simulink model "spot410"  (R2024b)
settings: Solver=ode4  StartTime=0.0  StopTime=tsim  FixedStep=baseRate  RelTol=1e-6  AbsTol=1e-6
values from neighbouring files (symbols this model uses):
  baseRate = paramEst(phase,coord).k1    [SpotEstimator.m]
  Gamma1_el = 0.12    [initSpotDefaultParam.m]
  Gamma1_sh = 0.005    [initSpotDefaultParam.m]
  Gamma1_wr = 0.025    [initSpotDefaultParam.m]
  Gamma2_el = 5    [initSpotDefaultParam.m]
  Gamma2_sh = 5    [initSpotDefaultParam.m]
  Gamma2_wr = 5    [initSpotDefaultParam.m]
  Gamma3_el = 10    [initSpotDefaultParam.m]
  Gamma3_sh = 40    [initSpotDefaultParam.m]
  Gamma3_wr = 40    [initSpotDefaultParam.m]
  Gamma4_el = 0.039    [initSpotDefaultParam.m]
  Gamma4_sh = 0.015    [initSpotDefaultParam.m]
  Gamma4_wr = 0.029    [initSpotDefaultParam.m]
  Gamma5_el = 800    [initSpotDefaultParam.m]
  Gamma5_sh = 800    [initSpotDefaultParam.m]
  Gamma5_wr = 800    [initSpotDefaultParam.m]
  Gamma6_el = 0.000001    (= 1e-06)    [initSpotDefaultParam.m]
  Gamma6_sh = 0.005    [initSpotDefaultParam.m]
  Gamma6_wr = 0.02    [initSpotDefaultParam.m]
  Kd_elarm = 0.8    [initSpotDefaultParam.m]
  Kd_sharm = 1.0    (= 1)    [initSpotDefaultParam.m]
  Kd_wrarm = 0.6    [initSpotDefaultParam.m]
  Kp_elarm = 1.2    [initSpotDefaultParam.m]
  Kp_sharm = 1.5    [initSpotDefaultParam.m]
  Kp_wrarm = 1.0    (= 1)    [initSpotDefaultParam.m]
  PWMFreq = 5    [initSpotDefaultParam.m]
  Tz_lim_elarm = .1    (= 0.1)    [initSpotDefaultParam.m]
  Tz_lim_sharm = .1    (= 0.1)    [initSpotDefaultParam.m]
  Tz_lim_wrarm = .1    (= 0.1)    [initSpotDefaultParam.m]
undefined symbols (not defined in the file or in its folder): a1, a2, a3, b0, b1, b2, b3, dataRate, DiscIntNeverNeededParam, drop_states_ARM, drop_states_BLACK, drop_states_BLUE, drop_states_RED, F_black_X_nominal, F_black_Y_nominal, F_blue_X_nominal, F_blue_Y_nominal, F_red_X_nominal, F_red_Y_nominal, F_thrusters_BLACK, F_thrusters_BLUE, F_thrusters_RED, home_states_BLACK, home_states_BLUE, home_states_RED, IBLACK, IBLUE, IDIST, IEE, init_states_BLACK, init_states_BLUE, init_states_RED, IPROX, IRED, K_BLACK, K_BLUE, K_RED, Kd_tb, Kd_tblue, Kd_tr, Kd_xb, Kd_xblue, Kd_xr, Kd_yb, Kd_yblue, Kd_yr, Kp_tb, Kp_tblue, Kp_tr, Kp_xb, Kp_xblue, Kp_xr, Kp_yb, Kp_yblue, Kp_yr, mBLACK, mBLUE, mDIST, mEE, mPROX ... (+21)
libraries: simulink x30, nvidiaSharedBlocks x19, MainLibrary x5, dspinverses x3, nvidiaIMUSensorslib x1
(part 4 of 8)

== system spot410/1 - Experiment Logic/Phase #3: Experiment/Sub-Phase #2  ==
  note: Experiment Logic (BLACK)
  note: Experiment Logic (Robotic Manipulator)
  note: Experiment Logic (BLUE)
  note: Experiment Logic (RED)
  note: Control Blocks
  Action Port : ActionPort  ActionPortLabel=elseif((u1 < u3 & u1 >= u2))
  Constant{11..12,14..15,18} (5 alike) : Constant  Value=0
  Constant4 : Constant  Value=2
  Constant5 : Constant  Value=2
  Constant6 : Constant
  Constant8 : Constant  Value=2
  Data Store Write1 : DataStoreWrite  DataStoreName=ARM_Path_Planner_Selection  IndexOptions=Index vector (dialog)  Indices=1  OutputSizes=1
  Data Store Write13 : DataStoreWrite  DataStoreName=ARM_Desired_States  IndexOptions=Index vector (dialog)  Indices=1  OutputSizes=1
  Data Store Write16 : DataStoreWrite  DataStoreName=BLUE_Control_Law_Enabler  IndexOptions=Index vector (dialog)  Indices=1  OutputSizes=1
  Data Store Write18 : DataStoreWrite  DataStoreName=BLUE_Desired_States  IndexOptions=Index vector (dialog)  Indices=1  OutputSizes=1
  Data Store Write2 : DataStoreWrite  DataStoreName=ARM_Control_Law_Enabler  IndexOptions=Index vector (dialog)  Indices=1  OutputSizes=1
  Data Store Write22 : DataStoreWrite  DataStoreName=BLUE_Path_Planner_Selection  IndexOptions=Index vector (dialog)  Indices=1  OutputSizes=1
  Data Store Write23 : DataStoreWrite  DataStoreName=BLACK_Path_Planner_Selection  IndexOptions=Index vector (dialog)  Indices=1  OutputSizes=1
  Data Store Write24 : DataStoreWrite  DataStoreName=RED_Path_Planner_Selection  IndexOptions=Index vector (dialog)  Indices=1  OutputSizes=1
  Data Store Write3 : DataStoreWrite  DataStoreName=RED_Control_Law_Enabler  IndexOptions=Index vector (dialog)  Indices=1  OutputSizes=1
  Data Store Write4 : DataStoreWrite  DataStoreName=BLACK_Control_Law_Enabler  IndexOptions=Index vector (dialog)  Indices=1  OutputSizes=1
  Data Store Write5 : DataStoreWrite  DataStoreName=BLACK_Desired_States  IndexOptions=Index vector (dialog)  Indices=1  OutputSizes=1
  Data Store Write7 : DataStoreWrite  DataStoreName=Float_State  IndexOptions=Index vector (dialog)  Indices=1  OutputSizes=1
  Data Store Write9 : DataStoreWrite  DataStoreName=RED_Desired_States  IndexOptions=Index vector (dialog)  Indices=1  OutputSizes=1
  Desired Joint Angles RED : Subsystem
  Desired Position BLACK : Subsystem
  Desired Position BLUE : Subsystem
  Desired Position RED : Subsystem
  wires:
  Desired Position RED/1(Target Array) -> Data Store Write9/1
  Desired Position BLACK/1(Target Array) -> Data Store Write5/1
  Desired Position BLUE/1(Target Array) -> Data Store Write18/1
  Constant12/1 -> Data Store Write1/1
  Constant18/1 -> Data Store Write2/1
  Constant6/1 -> Data Store Write7/1
  Constant15/1 -> Data Store Write22/1
  Constant14/1 -> Data Store Write23/1
  Constant5/1 -> Data Store Write3/1
  Constant11/1 -> Data Store Write24/1
  Constant8/1 -> Data Store Write16/1
  Constant4/1 -> Data Store Write4/1
  Desired Joint Angles RED/1(Target Array) -> Data Store Write13/1

== system spot410/1 - Experiment Logic/Phase #3: Experiment/Sub-Phase #3  ==
  note: Experiment Logic (BLACK)
  note: Experiment Logic (Robotic Manipulator)
  note: Experiment Logic (BLUE)
  note: Experiment Logic (RED)
  note: Control Blocks
  Action Port : ActionPort  ActionPortLabel=elseif((u1 < u4 & u1 >= u3))
  Constant{11..12,14..15,18} (5 alike) : Constant  Value=0
  Constant4 : Constant  Value=2
  Constant5 : Constant  Value=2
  Constant6 : Constant
  Constant8 : Constant  Value=2
  Data Store Write1 : DataStoreWrite  DataStoreName=ARM_Path_Planner_Selection  IndexOptions=Index vector (dialog)  Indices=1  OutputSizes=1
  Data Store Write13 : DataStoreWrite  DataStoreName=ARM_Desired_States  IndexOptions=Index vector (dialog)  Indices=1  OutputSizes=1
  Data Store Write16 : DataStoreWrite  DataStoreName=BLUE_Control_Law_Enabler  IndexOptions=Index vector (dialog)  Indices=1  OutputSizes=1
  Data Store Write18 : DataStoreWrite  DataStoreName=BLUE_Desired_States  IndexOptions=Index vector (dialog)  Indices=1  OutputSizes=1
  Data Store Write2 : DataStoreWrite  DataStoreName=ARM_Control_Law_Enabler  IndexOptions=Index vector (dialog)  Indices=1  OutputSizes=1
  Data Store Write22 : DataStoreWrite  DataStoreName=BLUE_Path_Planner_Selection  IndexOptions=Index vector (dialog)  Indices=1  OutputSizes=1
  Data Store Write23 : DataStoreWrite  DataStoreName=BLACK_Path_Planner_Selection  IndexOptions=Index vector (dialog)  Indices=1  OutputSizes=1
  Data Store Write24 : DataStoreWrite  DataStoreName=RED_Path_Planner_Selection  IndexOptions=Index vector (dialog)  Indices=1  OutputSizes=1
  Data Store Write3 : DataStoreWrite  DataStoreName=RED_Control_Law_Enabler  IndexOptions=Index vector (dialog)  Indices=1  OutputSizes=1
  Data Store Write4 : DataStoreWrite  DataStoreName=BLACK_Control_Law_Enabler  IndexOptions=Index vector (dialog)  Indices=1  OutputSizes=1
  Data Store Write5 : DataStoreWrite  DataStoreName=BLACK_Desired_States  IndexOptions=Index vector (dialog)  Indices=1  OutputSizes=1
  Data Store Write7 : DataStoreWrite  DataStoreName=Float_State  IndexOptions=Index vector (dialog)  Indices=1  OutputSizes=1
  Data Store Write9 : DataStoreWrite  DataStoreName=RED_Desired_States  IndexOptions=Index vector (dialog)  Indices=1  OutputSizes=1
  Desired Joint Angles RED : Subsystem
  Desired Position BLACK : Subsystem
  Desired Position BLUE : Subsystem
  Desired Position RED : Subsystem
  wires:
  Desired Position RED/1(Target Array) -> Data Store Write9/1
  Desired Position BLACK/1(Target Array) -> Data Store Write5/1
  Desired Position BLUE/1(Target Array) -> Data Store Write18/1
  Desired Joint Angles RED/1(Target Array) -> Data Store Write13/1
  Constant12/1 -> Data Store Write1/1
  Constant18/1 -> Data Store Write2/1
  Constant6/1 -> Data Store Write7/1
  Constant15/1 -> Data Store Write22/1
  Constant14/1 -> Data Store Write23/1
  Constant5/1 -> Data Store Write3/1
  Constant11/1 -> Data Store Write24/1
  Constant8/1 -> Data Store Write16/1
  Constant4/1 -> Data Store Write4/1

== system spot410/1 - Experiment Logic/Phase #3: Experiment/Sub-Phase #4 ==
  note: Experiment Logic (BLACK)
  note: Experiment Logic (Robotic Manipulator)
  note: Experiment Logic (BLUE)
  note: Experiment Logic (RED)
  note: Control Blocks
  Action Port : ActionPort  ActionPortLabel=elseif( (u1 < u5 & u1 >= u4))
  Constant{11..12,14..15,18} (5 alike) : Constant  Value=0
  Constant4 : Constant  Value=2
  Constant5 : Constant  Value=2
  Constant6 : Constant
  Constant8 : Constant  Value=2
  Data Store Write1 : DataStoreWrite  DataStoreName=ARM_Path_Planner_Selection  IndexOptions=Index vector (dialog)  Indices=1  OutputSizes=1
  Data Store Write13 : DataStoreWrite  DataStoreName=ARM_Desired_States  IndexOptions=Index vector (dialog)  Indices=1  OutputSizes=1
  Data Store Write16 : DataStoreWrite  DataStoreName=BLUE_Control_Law_Enabler  IndexOptions=Index vector (dialog)  Indices=1  OutputSizes=1
  Data Store Write18 : DataStoreWrite  DataStoreName=BLUE_Desired_States  IndexOptions=Index vector (dialog)  Indices=1  OutputSizes=1
  Data Store Write2 : DataStoreWrite  DataStoreName=ARM_Control_Law_Enabler  IndexOptions=Index vector (dialog)  Indices=1  OutputSizes=1
  Data Store Write22 : DataStoreWrite  DataStoreName=BLUE_Path_Planner_Selection  IndexOptions=Index vector (dialog)  Indices=1  OutputSizes=1
  Data Store Write23 : DataStoreWrite  DataStoreName=BLACK_Path_Planner_Selection  IndexOptions=Index vector (dialog)  Indices=1  OutputSizes=1
  Data Store Write24 : DataStoreWrite  DataStoreName=RED_Path_Planner_Selection  IndexOptions=Index vector (dialog)  Indices=1  OutputSizes=1
  Data Store Write3 : DataStoreWrite  DataStoreName=RED_Control_Law_Enabler  IndexOptions=Index vector (dialog)  Indices=1  OutputSizes=1
  Data Store Write4 : DataStoreWrite  DataStoreName=BLACK_Control_Law_Enabler  IndexOptions=Index vector (dialog)  Indices=1  OutputSizes=1
  Data Store Write5 : DataStoreWrite  DataStoreName=BLACK_Desired_States  IndexOptions=Index vector (dialog)  Indices=1  OutputSizes=1
  Data Store Write7 : DataStoreWrite  DataStoreName=Float_State  IndexOptions=Index vector (dialog)  Indices=1  OutputSizes=1
  Data Store Write9 : DataStoreWrite  DataStoreName=RED_Desired_States  IndexOptions=Index vector (dialog)  Indices=1  OutputSizes=1
  Desired Joint Angles RED : Subsystem
  Desired Position BLACK : Subsystem
  Desired Position BLUE : Subsystem
  Desired Position RED : Subsystem
  wires:
  Desired Position RED/1(Target Array) -> Data Store Write9/1
  Desired Position BLACK/1(Target Array) -> Data Store Write5/1
  Desired Position BLUE/1(Target Array) -> Data Store Write18/1
  Desired Joint Angles RED/1(Target Array) -> Data Store Write13/1
  Constant12/1 -> Data Store Write1/1
  Constant18/1 -> Data Store Write2/1
  Constant6/1 -> Data Store Write7/1
  Constant15/1 -> Data Store Write22/1
  Constant14/1 -> Data Store Write23/1
  Constant5/1 -> Data Store Write3/1
  Constant11/1 -> Data Store Write24/1
  Constant8/1 -> Data Store Write16/1
  Constant4/1 -> Data Store Write4/1

== system spot410/1 - Experiment Logic/Phase #4: Return Home/Desired Joint Angles RED ==
  Constant1 : Constant  Value=pi/2
  Constant2 : Constant  Value=0
  Constant3 : Constant  Value=pi/2
  Mux : Mux  Inputs=3
  Target Array : Outport
  wires:
  Mux/1 -> Target Array/1
  Constant3/1 -> Mux/1
  Constant1/1 -> Mux/2
  Constant2/1 -> Mux/3

== system spot410/1 - Experiment Logic/Phase #4: Return Home/Desired Position BLACK ==
  Desired States (BLACK) : Constant  Value=home_states_BLACK  SampleTime=-1
  Target Array : Outport
  wires:
  Desired States (BLACK)/1 -> Target Array/1

== system spot410/1 - Experiment Logic/Phase #4: Return Home/Desired Position BLUE ==
  Desired States (BLUE) : Constant  Value=home_states_BLUE  SampleTime=-1
  Target Array : Outport
  wires:
  Desired States (BLUE)/1 -> Target Array/1

== system spot410/1 - Experiment Logic/Phase #4: Return Home/Desired Position RED ==
  Constant2 : Constant  Value=home_states_RED
  Target Array : Outport
  wires:
  Constant2/1 -> Target Array/1

== system spot410/1 - Experiment Logic/Phase #5: Hold Home/Desired Joint Angles RED ==
  Constant1 : Constant  Value=pi/2
  Constant2 : Constant  Value=0
  Constant3 : Constant  Value=pi/2
  Mux : Mux  Inputs=3
  Target Array : Outport
  wires:
  Mux/1 -> Target Array/1
  Constant3/1 -> Mux/1
  Constant1/1 -> Mux/2
  Constant2/1 -> Mux/3

== system spot410/1 - Experiment Logic/Phase #5: Hold Home/Desired Position BLACK ==
  Desired States (BLACK) : Constant  Value=home_states_BLACK  SampleTime=-1
  Target Array : Outport
  wires:
  Desired States (BLACK)/1 -> Target Array/1

== system spot410/1 - Experiment Logic/Phase #5: Hold Home/Desired Position BLUE ==
  Desired States (BLUE) : Constant  Value=home_states_BLUE  SampleTime=-1
  Target Array : Outport
  wires:
  Desired States (BLUE)/1 -> Target Array/1

== system spot410/1 - Experiment Logic/Phase #5: Hold Home/Desired Position RED ==
  Constant2 : Constant  Value=home_states_RED
  Target Array : Outport
  wires:
  Constant2/1 -> Target Array/1

== system spot410/2 - Guidance/Custom PPL (ARM)/Desired Position ==
  Data Store Read : DataStoreRead  DataStoreName=ARM_Desired_States  IndexOptions=Index vector (dialog)  Indices=1  OutputSizes=1
  Position Array : Outport
  wires:
  Data Store Read/1 -> Position Array/1

== system spot410/2 - Guidance/Custom PPL (BLACK)/Desired Position ==
  BLACK_Px : DataStoreRead  DataStoreName=BLACK_Desired_States  IndexOptions=Index vector (dialog)  Indices=1  OutputSizes=1
  Position Array : Outport
  wires:
  BLACK_Px/1 -> Position Array/1

== system spot410/2 - Guidance/Custom PPL (BLUE)/Desired Position ==
  Data Store Read4 : DataStoreRead  DataStoreName=BLUE_Desired_States  IndexOptions=Index vector (dialog)  Indices=1  OutputSizes=1
  Position Array : Outport
  wires:
  Data Store Read4/1 -> Position Array/1

== system spot410/2 - Guidance/Custom PPL (RED)/Desired Position ==
  RED_Px : DataStoreRead  DataStoreName=RED_Desired_States  IndexOptions=Index vector (dialog)  Indices=1  OutputSizes=1
  Position Array : Outport
  wires:
  RED_Px/1 -> Position Array/1

== system spot410/2 - Guidance/Default APF PPL (BLACK)/Current Position RED ==
  Demux : Demux  Outputs=[3,6]
  RED_Px : DataStoreRead  DataStoreName=BLACK_Measured_States  IndexOptions=Index vector (dialog)  Indices=1  OutputSizes=1
  Terminator : Terminator
  Position Array : Outport
  wires:
  RED_Px/1 -> Demux/1
  Demux/1 -> Position Array/1
  Demux/2 -> Terminator/1

== system spot410/2 - Guidance/Default APF PPL (BLACK)/Obstacles ==
  Current Position BLUE : Subsystem
  Current Position RED : Subsystem
  Matrix Concatenate : Concatenate  Mode=Multidimensional array
  Obstacle Positions : Outport
  wires:
  Current Position RED/1(Position Array) -> Matrix Concatenate/2
  Current Position BLUE/1(Position Array) -> Matrix Concatenate/1
  Matrix Concatenate/1 -> Obstacle Positions/1

== system spot410/2 - Guidance/Default APF PPL (RED)/Current Position RED ==
  Demux : Demux  Outputs=[3,6]
  RED_Px : DataStoreRead  DataStoreName=RED_Measured_States  IndexOptions=Index vector (dialog)  Indices=1  OutputSizes=1
  Terminator : Terminator
  Position Array : Outport
  wires:
  RED_Px/1 -> Demux/1
  Demux/1 -> Position Array/1
  Demux/2 -> Terminator/1

== system spot410/2 - Guidance/Default APF PPL (RED)/Obstacles ==
  Current Position BLACK : Subsystem
  Current Position BLUE : Subsystem
  Matrix Concatenate : Concatenate  Mode=Multidimensional array
  Obstacle Positions : Outport
  wires:
  Current Position BLACK/1(Position Array) -> Matrix Concatenate/2
  Current Position BLUE/1(Position Array) -> Matrix Concatenate/1
  Matrix Concatenate/1 -> Obstacle Positions/1

== system spot410/2 - Guidance/Disable PPL (ARM)/Desired Position ==
  Data Store Read : DataStoreRead  DataStoreName=ARM_Desired_States  IndexOptions=Index vector (dialog)  Indices=1  OutputSizes=1
  Position Array : Outport
  wires:
  Data Store Read/1 -> Position Array/1

== system spot410/2 - Guidance/Disable PPL (BLACK)/Desired Position ==
  BLACK_Px : DataStoreRead  DataStoreName=BLACK_Desired_States  IndexOptions=Index vector (dialog)  Indices=1  OutputSizes=1
  Position Array : Outport
  wires:
  BLACK_Px/1 -> Position Array/1

== system spot410/2 - Guidance/Disable PPL (BLUE)/Desired Position ==
  Data Store Read4 : DataStoreRead  DataStoreName=BLUE_Desired_States  IndexOptions=Index vector (dialog)  Indices=1  OutputSizes=1
  Position Array : Outport
  wires:
  Data Store Read4/1 -> Position Array/1

== system spot410/2 - Guidance/Disable PPL (RED)/Desired Position ==
  RED_Px : DataStoreRead  DataStoreName=RED_Desired_States  IndexOptions=Index vector (dialog)  Indices=1  OutputSizes=1
  Position Array : Outport
  wires:
  RED_Px/1 -> Position Array/1

== system spot410/3 - Control/Default LQR Control (BLACK)/Calculate Error ==
  Desired Attitude : Inport
  Measured Attitude : Inport  Port=2
  MATLAB Function : MATLAB Function  TreatAsAtomicUnit=on
  Attitude Error : Outport
  wires:
  MATLAB Function/1(Rz_error) -> Attitude Error/1
  Desired Attitude/1 -> MATLAB Function/1(Rz_path)
  Measured Attitude/1 -> MATLAB Function/2(Rz_measured)

== system spot410/3 - Control/Default LQR Control (BLUE)/Calculate Error ==
  Desired Attitude : Inport
  Measured Attitude : Inport  Port=2
  MATLAB Function : MATLAB Function  TreatAsAtomicUnit=on
  Attitude Error : Outport
  wires:
  MATLAB Function/1(Rz_error) -> Attitude Error/1
  Desired Attitude/1 -> MATLAB Function/1(Rz_path)
  Measured Attitude/1 -> MATLAB Function/2(Rz_measured)

== system spot410/3 - Control/Default LQR Control (RED)/Calculate Error ==
  Desired Attitude : Inport
  Measured Attitude : Inport  Port=2
  MATLAB Function : MATLAB Function  TreatAsAtomicUnit=on
  Attitude Error : Outport
  wires:
  MATLAB Function/1(Rz_error) -> Attitude Error/1
  Desired Attitude/1 -> MATLAB Function/1(Rz_path)
  Measured Attitude/1 -> MATLAB Function/2(Rz_measured)

== system spot410/3 - Control/Default PD (ARM)/Passthrough for Experiment ==
  q1_desired : Inport
  q2_desired : Inport  Port=2
  q3_desired : Inport  Port=3
  Action Port : ActionPort  ActionPortLabel=else
  q1_command : Outport
  q2_command : Outport  Port=2
  q3_command : Outport  Port=3
  wires:
  q3_desired/1 -> q3_command/1
  q1_desired/1 -> q1_command/1
  q2_desired/1 -> q2_command/1

== system spot410/3 - Control/Default PD (ARM)/Simulated Position Controller ==
  q1_desired : Inport
  q2_desired : Inport  Port=2
  q3_desired : Inport  Port=3
  Action Port : ActionPort  ActionPortLabel=if(u1 == 1)
  Custom Discrete PD (Elbow) : Subsystem
  Custom Discrete PD (Shoulder) : Subsystem
  Custom Discrete PD (Wrist) : Subsystem
  Data Store Read2 : DataStoreRead  DataStoreName=ARM_Measured_States  IndexOptions=Index vector (dialog)  Indices=1  OutputSizes=1
  Demux : Demux  Outputs=[1,1,1,3]
  Saturation : Saturate  UpperLimit=Tz_lim_sharm  LowerLimit=-Tz_lim_sharm
  Saturation1 : Saturate  UpperLimit=Tz_lim_elarm  LowerLimit=-Tz_lim_elarm
  Saturation3 : Saturate  UpperLimit=Tz_lim_wrarm  LowerLimit=-Tz_lim_wrarm
  Subtract2 : Sum  Inputs=+-
  Subtract3 : Sum  Inputs=+-
  Subtract4 : Sum  Inputs=+-
  Terminator : Terminator
  q1_command : Outport
  q2_command : Outport  Port=2
  q3_command : Outport  Port=3
  wires:
  Saturation3/1 -> q3_command/1
  Subtract4/1 -> Custom Discrete PD (Wrist)/1(ey)
  Custom Discrete PD (Shoulder)/1(Fx) -> Saturation/1
  Custom Discrete PD (Elbow)/1(Fy) -> Saturation1/1
  Saturation/1 -> q1_command/1
  Subtract2/1 -> Custom Discrete PD (Shoulder)/1(ex)
  Saturation1/1 -> q2_command/1
  Custom Discrete PD (Wrist)/1(Fy) -> Saturation3/1
  Subtract3/1 -> Custom Discrete PD (Elbow)/1(ey)
  Demux/1 -> Subtract2/2
  Demux/2 -> Subtract3/2
  Demux/3 -> Subtract4/2
  q1_desired/1 -> Subtract2/1
  q2_desired/1 -> Subtract3/1
  q3_desired/1 -> Subtract4/1
  Data Store Read2/1 -> Demux/1
  Demux/4 -> Terminator/1

== system spot410/3 - Control/Default PD Control (BLACK)/Calculate Error ==
  Desired Attitude : Inport
  Measured Attitude : Inport  Port=2
  MATLAB Function : MATLAB Function  TreatAsAtomicUnit=on
  Attitude Error : Outport
  wires:
  MATLAB Function/1(Rz_error) -> Attitude Error/1
  Desired Attitude/1 -> MATLAB Function/1(Rz_path)
  Measured Attitude/1 -> MATLAB Function/2(Rz_measured)

== system spot410/3 - Control/Default PD Control (BLUE)/Calculate Error ==
  Desired Attitude : Inport
  Measured Attitude : Inport  Port=2
  MATLAB Function : MATLAB Function  TreatAsAtomicUnit=on
  Attitude Error : Outport
  wires:
  MATLAB Function/1(Rz_error) -> Attitude Error/1
  Desired Attitude/1 -> MATLAB Function/1(Rz_path)
  Measured Attitude/1 -> MATLAB Function/2(Rz_measured)

== system spot410/3 - Control/Default PD Control (RED)/Calculate Error ==
  Desired Attitude : Inport
  Measured Attitude : Inport  Port=2
  MATLAB Function : MATLAB Function  TreatAsAtomicUnit=on
  Attitude Error : Outport
  wires:
  MATLAB Function/1(Rz_error) -> Attitude Error/1
  Desired Attitude/1 -> MATLAB Function/1(Rz_path)
  Measured Attitude/1 -> MATLAB Function/2(Rz_measured)

== system spot410/PhaseSpace Camera Code/Use Hardware to Obtain States/Receive and Process Phasespace Data ==
  "Adjust Time " : Subsystem
  Check for Sychronization : Subsystem
  Clock : Clock
  Demux2 : Demux  Outputs=[1,18]
  Mux : Mux  Inputs=2
  Receive PhaseSpace Data : nvidiaSharedBlocks/UDP Receive  localURL='0.0.0.0'  localPort=31534  remoteURL='0.0.0.0'  remotePort=-1  recvBufferSize=8192  signalDatatype=double  dims=19  isVarSize=off  showBlockingTime=off  blockingTime=0  sampletime=-1  blockPlatform=NVIDIA
  Reshape : Reshape  OutputDimensionality=Customize  OutputDimensions=[19,1]
  Terminator : Terminator
  PhaseSpace Data : Outport
  PhaseSpace Clock : Outport  Port=2
  wires:
  Check for Sychronization/1(StartClock) -> "Adjust Time "/1(ClockStart)
  Reshape/1 -> Demux2/1
  "Adjust Time "/1(ClockAdjusted) -> Mux/1
  Demux2/2 -> Mux/2
  Mux/1 -> PhaseSpace Data/1
  Receive PhaseSpace Data/2 -> Terminator/1
  Receive PhaseSpace Data/1 -> Reshape/1
  Clock/1 -> "Adjust Time "/2(ClockRaw)
  Demux2/1 -> PhaseSpace Clock/1

== system spot410/PhaseSpace Camera Code/Use Hardware to Obtain States/Store BLACK Data ==
  note: Store BLACK Positions and Velocities
  BLACK Data : Inport
  BLACK Velocities : Inport  Port=2
  PS Clock : Inport  Port=3
  Calculate True Time Step : Subsystem
      settings: PortSchema="{\"entries\":[{\"content\":{\"sides\":[{\"content\":{\"connectorIds\":[\"In1\"]},\"type\":\"ConnectorPlacement.EquallySpacedRectSide\",\"uuid\":\"62932c5c-f2a7-44c8-96b4-4a75bab3a126\"},{\"content\":{\"connectorIds\":[\"Out1\"],\"side\":\"RIGHT\"},\"type\":\"ConnectorPlacement.EquallySpacedRectSide\",\"uuid\":\"82b3b717-2171-4047-b0df-3cd41cf9dfc7\"},{\"content\":{\"side\":\"TOP\"},\"type\":\"ConnectorPlacement.EquallySpacedRectSide\",\"uuid\":\"a142272a-a0ff-4882-8a2d-4633b3c7e02f\"},{\"content\":{\"connectorIds\":[\"In2\"],\"side\":\"BOTTOM\"},\"type\":\"ConnectorPlacement.EquallySpacedRectSide\",\"uuid\":\"b1e1ff4c-66d6-488f-92fb-77f76780833b\"}]},\"type\":\"ConnectorPlacement.EquallySpacedConnector\",\"uuid\":\"98c51868-8a10-4b52-aae4-56f6042c65c4\"}],\"packageUris\":[\"http://schema.mathworks.com/mf0/Connector/R2020b\"],\"version\":\"1.0\"}"
  Convert BLACKVX from [mm] to [m] : Gain  Gain=1/1000
  Convert BLACKVY from [mm] to [m] : Gain  Gain=1/1000
  Convert BLAX from [mm] to [m] : Gain  Gain=1/1000
  Convert BLAY from [mm] to [m] : Gain  Gain=1/1000
  Demux : Demux  Outputs=3
  Demux2 : Demux  Outputs=3
  Demux3 : Demux  Outputs=3
  Mux{1..4} (4 alike) : Mux  Inputs=3
  RED_Px7 : DataStoreWrite  DataStoreName=BLACK_Measured_States  IndexOptions=Index vector (dialog)  Indices=1  OutputSizes=1
  Reshape : Reshape  OutputDimensionality=Column vector (2-D)
  Subsystem1 : Subsystem
  Subsystem2 : Subsystem
  Wrap : Subsystem
  wires:
  Demux3/1 -> Convert BLAX from [mm] to [m]/1
  Demux3/2 -> Convert BLAY from [mm] to [m]/1
  BLACK Data/1 -> Demux3/1
  Demux/3 -> Wrap/1(Unwrapped Angle)
  Reshape/1 -> Subsystem1/2(y)
  Demux/1 -> Mux1/1
  Convert BLAY from [mm] to [m]/1 -> Mux3/2
  Calculate True Time Step/1(dt_out) -> Subsystem2/1(dt), Subsystem1/1(dt)
  Mux3/1 -> Subsystem2/2(y), Demux/1, Calculate True Time Step/2(Data)
  Wrap/1(Wrapped Angle) -> Mux1/3
  Convert BLAX from [mm] to [m]/1 -> Mux3/1
  Mux2/1 -> RED_Px7/1
  Demux/2 -> Mux1/2
  Subsystem2/1(dy/dt) -> Reshape/1
  PS Clock/1 -> Calculate True Time Step/1(Time)
  Demux3/3 -> Mux3/3
  Mux1/1 -> Mux2/1
  Subsystem1/1(dy/dt) -> Mux2/3
  BLACK Velocities/1 -> Demux2/1
  Demux2/3 -> Mux4/3
  Convert BLACKVX from [mm] to [m]/1 -> Mux4/1
  Convert BLACKVY from [mm] to [m]/1 -> Mux4/2
  Mux4/1 -> Mux2/2
  Demux2/2 -> Convert BLACKVY from [mm] to [m]/1
  Demux2/1 -> Convert BLACKVX from [mm] to [m]/1

== system spot410/PhaseSpace Camera Code/Use Hardware to Obtain States/Store BLUE Data ==
  note: Store BLUE Positions and Velocities
  BLUE Data : Inport
  BLUE Velocities : Inport  Port=2
  PS Clock : Inport  Port=3
  Calculate True Time Step : Subsystem
      settings: PortSchema="{\"entries\":[{\"content\":{\"sides\":[{\"content\":{\"connectorIds\":[\"In1\"]},\"type\":\"ConnectorPlacement.EquallySpacedRectSide\",\"uuid\":\"62932c5c-f2a7-44c8-96b4-4a75bab3a126\"},{\"content\":{\"connectorIds\":[\"Out1\"],\"side\":\"RIGHT\"},\"type\":\"ConnectorPlacement.EquallySpacedRectSide\",\"uuid\":\"82b3b717-2171-4047-b0df-3cd41cf9dfc7\"},{\"content\":{\"side\":\"TOP\"},\"type\":\"ConnectorPlacement.EquallySpacedRectSide\",\"uuid\":\"a142272a-a0ff-4882-8a2d-4633b3c7e02f\"},{\"content\":{\"connectorIds\":[\"In2\"],\"side\":\"BOTTOM\"},\"type\":\"ConnectorPlacement.EquallySpacedRectSide\",\"uuid\":\"b1e1ff4c-66d6-488f-92fb-77f76780833b\"}]},\"type\":\"ConnectorPlacement.EquallySpacedConnector\",\"uuid\":\"98c51868-8a10-4b52-aae4-56f6042c65c4\"}],\"packageUris\":[\"http://schema.mathworks.com/mf0/Connector/R2020b\"],\"version\":\"1.0\"}"
  Convert BLUEVX from [mm] to [m] : Gain  Gain=1/1000
  Convert BLUEVY from [mm] to [m] : Gain  Gain=1/1000
  Convert BLUX from [mm] to [m] : Gain  Gain=1/1000
  Convert BLUY from [mm] to [m] : Gain  Gain=1/1000
  Demux : Demux  Outputs=3
  Demux2 : Demux  Outputs=3
  Demux5 : Demux  Outputs=3
  Mux{1..4} (4 alike) : Mux  Inputs=3
  RED_Px7 : DataStoreWrite  DataStoreName=BLUE_Measured_States  IndexOptions=Index vector (dialog)  Indices=1  OutputSizes=1
  Reshape : Reshape  OutputDimensionality=Column vector (2-D)
  Subsystem1 : Subsystem
  Subsystem2 : Subsystem
  Wrap : Subsystem
  wires:
  Demux5/2 -> Convert BLUY from [mm] to [m]/1
  Demux5/1 -> Convert BLUX from [mm] to [m]/1
  BLUE Data/1 -> Demux5/1
  Calculate True Time Step/1(dt_out) -> Subsystem2/1(dt), Subsystem1/1(dt)
  Demux/2 -> Mux1/2
  Demux/1 -> Mux1/1
  Subsystem2/1(dy/dt) -> Reshape/1
  Mux3/1 -> Subsystem2/2(y), Demux/1, Calculate True Time Step/2(Data)
  Demux/3 -> Wrap/1(Unwrapped Angle)
  Reshape/1 -> Subsystem1/2(y)
  Wrap/1(Wrapped Angle) -> Mux1/3
  Mux2/1 -> RED_Px7/1
  Convert BLUY from [mm] to [m]/1 -> Mux3/2
  Convert BLUX from [mm] to [m]/1 -> Mux3/1
  Demux5/3 -> Mux3/3
  PS Clock/1 -> Calculate True Time Step/1(Time)
  Mux1/1 -> Mux2/1
  Subsystem1/1(dy/dt) -> Mux2/3
  Demux2/1 -> Convert BLUEVX from [mm] to [m]/1
  Convert BLUEVY from [mm] to [m]/1 -> Mux4/2
  BLUE Velocities/1 -> Demux2/1
  Demux2/2 -> Convert BLUEVY from [mm] to [m]/1
  Mux4/1 -> Mux2/2
  Demux2/3 -> Mux4/3
  Convert BLUEVX from [mm] to [m]/1 -> Mux4/1

== system spot410/PhaseSpace Camera Code/Use Hardware to Obtain States/Store RED Data ==
  note: Store RED Position and Velocity Data
  RED Data : Inport
  RED Velocities : Inport  Port=2
  PS Clock : Inport  Port=3
  Calculate True Time Step : Subsystem
      settings: PortSchema="{\"entries\":[{\"content\":{\"sides\":[{\"content\":{\"connectorIds\":[\"In1\"]},\"type\":\"ConnectorPlacement.EquallySpacedRectSide\",\"uuid\":\"62932c5c-f2a7-44c8-96b4-4a75bab3a126\"},{\"content\":{\"connectorIds\":[\"Out1\"],\"side\":\"RIGHT\"},\"type\":\"ConnectorPlacement.EquallySpacedRectSide\",\"uuid\":\"82b3b717-2171-4047-b0df-3cd41cf9dfc7\"},{\"content\":{\"side\":\"TOP\"},\"type\":\"ConnectorPlacement.EquallySpacedRectSide\",\"uuid\":\"a142272a-a0ff-4882-8a2d-4633b3c7e02f\"},{\"content\":{\"connectorIds\":[\"In2\"],\"side\":\"BOTTOM\"},\"type\":\"ConnectorPlacement.EquallySpacedRectSide\",\"uuid\":\"b1e1ff4c-66d6-488f-92fb-77f76780833b\"}]},\"type\":\"ConnectorPlacement.EquallySpacedConnector\",\"uuid\":\"98c51868-8a10-4b52-aae4-56f6042c65c4\"}],\"packageUris\":[\"http://schema.mathworks.com/mf0/Connector/R2020b\"],\"version\":\"1.0\"}"
  Convert REDVX from [mm] to [m] : Gain  Gain=1/1000
  Convert REDVY from [mm] to [m] : Gain  Gain=1/1000
  Convert REDX from [mm] to [m] : Gain  Gain=1/1000
  Convert REDY from [mm] to [m] : Gain  Gain=1/1000
  Demux : Demux  Outputs=3
  Demux1 : Demux
  Demux2 : Demux  Outputs=3
  Mux{1..4} (4 alike) : Mux  Inputs=3
  RED_Px7 : DataStoreWrite  DataStoreName=RED_Measured_States  IndexOptions=Index vector (dialog)  Indices=1  OutputSizes=1
  Reshape : Reshape  OutputDimensionality=Column vector (2-D)
  Subsystem1 : Subsystem
  Subsystem2 : Subsystem
  Universal_Time : DataStoreWrite  DataStoreName=Univ_Time  IndexOptions=Index vector (dialog)  Indices=1  OutputSizes=1
  Wrap : Subsystem
  wires:
  Demux1/2 -> Convert REDX from [mm] to [m]/1
  Demux1/3 -> Convert REDY from [mm] to [m]/1
  RED Data/1 -> Demux1/1
  Demux1/4 -> Mux3/3
  Demux1/1 -> Universal_Time/1
  Mux2/1 -> RED_Px7/1
  Reshape/1 -> Subsystem1/2(y)
  Wrap/1(Wrapped Angle) -> Mux1/3
  Demux/3 -> Wrap/1(Unwrapped Angle)
  Demux/1 -> Mux1/1
  Subsystem2/1(dy/dt) -> Reshape/1
  Mux3/1 -> Subsystem2/2(y), Demux/1, Calculate True Time Step/2(Data)
  Demux/2 -> Mux1/2
  Convert REDX from [mm] to [m]/1 -> Mux3/1
  Convert REDY from [mm] to [m]/1 -> Mux3/2
  Calculate True Time Step/1(dt_out) -> Subsystem2/1(dt), Subsystem1/1(dt)
  Mux1/1 -> Mux2/1
  Subsystem1/1(dy/dt) -> Mux2/3
  Convert REDVX from [mm] to [m]/1 -> Mux4/1
  Convert REDVY from [mm] to [m]/1 -> Mux4/2
  Demux2/1 -> Convert REDVX from [mm] to [m]/1
  Demux2/2 -> Convert REDVY from [mm] to [m]/1
  Demux2/3 -> Mux4/3
  RED Velocities/1 -> Demux2/1
  Mux4/1 -> Mux2/2
  PS Clock/1 -> Calculate True Time Step/1(Time)

== system spot410/Simulate Plant Dynamics/BLACK Dynamics/Calculated & Store Measured States ==
  y : Inport
  dt : Inport  Port=2
  Demux : Demux  Outputs=3
  Measured States for BLACK : DataStoreWrite  DataStoreName=BLACK_Measured_States  IndexOptions=Index vector (dialog)  Indices=1  OutputSizes=1
  Mux1 : Mux  Inputs=3
  Mux2 : Mux  Inputs=3
  Reshape : Reshape  OutputDimensionality=Column vector (2-D)
  Subsystem1 : Subsystem
  Subsystem2 : Subsystem
  Wrap : Subsystem
  wires:
  Demux/1 -> Mux1/1
  Wrap/1(Wrapped Angle) -> Mux1/3
  Demux/3 -> Wrap/1(Unwrapped Angle)
  Demux/2 -> Mux1/2
  Mux2/1 -> Measured States for BLACK/1
  Reshape/1 -> Subsystem1/2(y)
  Subsystem2/1(dy/dt) -> Mux2/2, Reshape/1
  y/1 -> Subsystem2/2(y), Demux/1
  Mux1/1 -> Mux2/1
  Subsystem1/1(dy/dt) -> Mux2/3
  dt/1 -> Subsystem1/1(dt), Subsystem2/1(dt)

== system spot410/Simulate Plant Dynamics/BLACK Dynamics/Calculated & Store True States ==
  y : Inport
  Demux : Demux  Outputs=3
  Discrete Derivative : simulink/Discrete/Discrete Derivative  gainval=1.0  ICPrevScaledInput=0.0  OutMin=[]  OutMax=[]  OutDataType=fixdt(1, 16)  OutScaling=2^-10  DoSatur=off
  Discrete Derivative1 : simulink/Discrete/Discrete Derivative  gainval=1.0  ICPrevScaledInput=0.0  OutMin=[]  OutMax=[]  OutDataType=fixdt(1, 16)  OutScaling=2^-10  DoSatur=off
  Mux1 : Mux  Inputs=3
  Mux2 : Mux  Inputs=3
  True States for BLACK : DataStoreWrite  DataStoreName=BLACK_True_States  IndexOptions=Index vector (dialog)  Indices=1  OutputSizes=1
  Wrap : Subsystem
  wires:
  Demux/1 -> Mux1/1
  Wrap/1(Wrapped Angle) -> Mux1/3
  Demux/3 -> Wrap/1(Unwrapped Angle)
  Demux/2 -> Mux1/2
  Mux2/1 -> True States for BLACK/1
  y/1 -> Discrete Derivative/1, Demux/1
  Discrete Derivative/1 -> Mux2/2, Discrete Derivative1/1
  Mux1/1 -> Mux2/1
  Discrete Derivative1/1 -> Mux2/3

== system spot410/Simulate Plant Dynamics/BLACK Dynamics/Data @ Measurement Rate ==
  Data Input : Inport
  Calculate True Time Step : Subsystem
  Constant1 : Constant  Value=dataRate
  Constant2 : Constant  Value=0
  Data Store Read : DataStoreRead  DataStoreName=Univ_Time  IndexOptions=Index vector (dialog)  Indices=1  OutputSizes=1
  Delay : Delay  DelayLength=1
  Enabled Subsystem : Subsystem  TreatAsAtomicUnit=on
  Enabled Subsystem1 : Subsystem  TreatAsAtomicUnit=on
  Relational Operator1 : RelationalOperator  OutDataTypeStr=boolean  RndMeth=Simplest  InputSameDT=off
  Relational Operator2 : RelationalOperator  Operator===  OutDataTypeStr=boolean  RndMeth=Simplest  InputSameDT=off
  Subtract : Sum  Inputs=+-
  Data Held : Outport
  Time Step : Outport  Port=2
  wires:
  Data Input/1 -> Enabled Subsystem1/1(ThrustPer_Final)
  Subtract/1 -> Relational Operator2/1, Delay/1
  Relational Operator2/1 -> Enabled Subsystem1/Enable
  Relational Operator1/1 -> Enabled Subsystem/Enable
  Constant1/1 -> Calculate True Time Step/3(Rate), Relational Operator1/2
  Constant2/1 -> Relational Operator2/2
  Enabled Subsystem/1(Out1) -> Calculate True Time Step/2(Time), Subtract/2
  Delay/1 -> Relational Operator1/1
  Data Store Read/1 -> Enabled Subsystem/1(In1), Subtract/1
  Enabled Subsystem1/1(Out1) -> Calculate True Time Step/1(Data), Data Held/1
  Calculate True Time Step/1(dt_out) -> Time Step/1

== system spot410/Simulate Plant Dynamics/BLACK Dynamics/Dynamics Model for BLACK ==
  control_inputs : Inport
  Acceleration to Velocity : DiscreteIntegrator  IntegratorMethod=Integration: Backward Euler  SampleTime=-1  ICPrevOutput=DiscIntNeverNeededParam  ICPrevScaledInput=DiscIntNeverNeededParam
  MATLAB Function : MATLAB Function  TreatAsAtomicUnit=on
  Velocity to Position : DiscreteIntegrator  IntegratorMethod=Integration: Backward Euler  InitialCondition=drop_states_BLACK  SampleTime=-1  ICPrevOutput=DiscIntNeverNeededParam  ICPrevScaledInput=DiscIntNeverNeededParam
  states : Outport  VectorParamsAs1DForOutWhenUnconnected=off
  wires:
  control_inputs/1 -> MATLAB Function/1(control_inputs)
  MATLAB Function/1(x_ddot) -> Acceleration to Velocity/1
  Acceleration to Velocity/1 -> Velocity to Position/1
  Velocity to Position/1 -> states/1

== system spot410/Simulate Plant Dynamics/BLUE Dynamics/BLUE  Dynamics Model ==
  control_inputs : Inport
  Acceleration to Velocity : DiscreteIntegrator  IntegratorMethod=Integration: Backward Euler  SampleTime=-1  ICPrevOutput=DiscIntNeverNeededParam  ICPrevScaledInput=DiscIntNeverNeededParam
  MATLAB Function : MATLAB Function  TreatAsAtomicUnit=on
  Velocity to Position : DiscreteIntegrator  IntegratorMethod=Integration: Backward Euler  InitialCondition=drop_states_BLUE  SampleTime=-1  ICPrevOutput=DiscIntNeverNeededParam  ICPrevScaledInput=DiscIntNeverNeededParam
  states : Outport  VectorParamsAs1DForOutWhenUnconnected=off
  wires:
  control_inputs/1 -> MATLAB Function/1(control_inputs)
  MATLAB Function/1(x_ddot) -> Acceleration to Velocity/1
  Acceleration to Velocity/1 -> Velocity to Position/1
  Velocity to Position/1 -> states/1

== system spot410/Simulate Plant Dynamics/BLUE Dynamics/Calculated & Store Measured States ==
  y : Inport
  dt : Inport  Port=2
  Demux : Demux  Outputs=3
  Measured States for BLUE : DataStoreWrite  DataStoreName=BLUE_Measured_States  IndexOptions=Index vector (dialog)  Indices=1  OutputSizes=1
  Mux1 : Mux  Inputs=3
  Mux2 : Mux  Inputs=3
  Reshape : Reshape  OutputDimensionality=Column vector (2-D)
  Subsystem1 : Subsystem
  Subsystem2 : Subsystem
  Wrap : Subsystem
  wires:
  Demux/1 -> Mux1/1
  Wrap/1(Wrapped Angle) -> Mux1/3
  Demux/3 -> Wrap/1(Unwrapped Angle)
  Demux/2 -> Mux1/2
  Mux2/1 -> Measured States for BLUE/1
  Reshape/1 -> Subsystem1/2(y)
  Subsystem2/1(dy/dt) -> Mux2/2, Reshape/1
  y/1 -> Subsystem2/2(y), Demux/1
  dt/1 -> Subsystem1/1(dt), Subsystem2/1(dt)
  Subsystem1/1(dy/dt) -> Mux2/3
  Mux1/1 -> Mux2/1

== system spot410/Simulate Plant Dynamics/BLUE Dynamics/Calculated & Store True States ==
  y : Inport
  Demux : Demux  Outputs=3
  Discrete Derivative : simulink/Discrete/Discrete Derivative  gainval=1.0  ICPrevScaledInput=0.0  OutMin=[]  OutMax=[]  OutDataType=fixdt(1, 16)  OutScaling=2^-10  DoSatur=off
  Discrete Derivative1 : simulink/Discrete/Discrete Derivative  gainval=1.0  ICPrevScaledInput=0.0  OutMin=[]  OutMax=[]  OutDataType=fixdt(1, 16)  OutScaling=2^-10  DoSatur=off
  Mux1 : Mux  Inputs=3
  Mux2 : Mux  Inputs=3
  True States for BLUE : DataStoreWrite  DataStoreName=BLUE_True_States  IndexOptions=Index vector (dialog)  Indices=1  OutputSizes=1
  Wrap : Subsystem
  wires:
  Demux/1 -> Mux1/1
  Wrap/1(Wrapped Angle) -> Mux1/3
  Demux/3 -> Wrap/1(Unwrapped Angle)
  Demux/2 -> Mux1/2
  Mux2/1 -> True States for BLUE/1
  Mux1/1 -> Mux2/1
  y/1 -> Discrete Derivative/1, Demux/1
  Discrete Derivative/1 -> Discrete Derivative1/1, Mux2/2
  Discrete Derivative1/1 -> Mux2/3

== system spot410/Simulate Plant Dynamics/BLUE Dynamics/Data @ Measurement Rate ==
  Data Input : Inport
  Calculate True Time Step : Subsystem
  Constant1 : Constant  Value=dataRate
  Constant2 : Constant  Value=0
  Data Store Read : DataStoreRead  DataStoreName=Univ_Time  IndexOptions=Index vector (dialog)  Indices=1  OutputSizes=1
  Delay : Delay  DelayLength=1
  Enabled Subsystem : Subsystem  TreatAsAtomicUnit=on
  Enabled Subsystem1 : Subsystem  TreatAsAtomicUnit=on
  Relational Operator1 : RelationalOperator  OutDataTypeStr=boolean  RndMeth=Simplest  InputSameDT=off
  Relational Operator2 : RelationalOperator  Operator===  OutDataTypeStr=boolean  RndMeth=Simplest  InputSameDT=off
  Subtract : Sum  Inputs=+-
  Data Held : Outport
  Time Step : Outport  Port=2
  wires:
  Data Input/1 -> Enabled Subsystem1/1(ThrustPer_Final)
  Subtract/1 -> Relational Operator2/1, Delay/1
  Relational Operator2/1 -> Enabled Subsystem1/Enable
  Relational Operator1/1 -> Enabled Subsystem/Enable
  Constant1/1 -> Calculate True Time Step/3(Rate), Relational Operator1/2
  Constant2/1 -> Relational Operator2/2
  Enabled Subsystem/1(Out1) -> Calculate True Time Step/2(Time), Subtract/2
  Delay/1 -> Relational Operator1/1
  Data Store Read/1 -> Enabled Subsystem/1(In1), Subtract/1
  Enabled Subsystem1/1(Out1) -> Calculate True Time Step/1(Data), Data Held/1
  Calculate True Time Step/1(dt_out) -> Time Step/1

== system spot410/Simulate Plant Dynamics/RED and ARM Dynamics/RED + ARM ==
  Action Port : ActionPort  ActionPortLabel=if(u1 == 4 | u1 == 5 | u1 == 10 | u1 == 11)
  Acceleration to Velocity : DiscreteIntegrator  IntegratorMethod=Integration: Backward Euler  InitialCondition=[0;0;0;0;0;0]  SampleTime=-1  ICPrevOutput=DiscIntNeverNeededParam  ICPrevScaledInput=DiscIntNeverNeededParam
  Add Noise : RandomNumber  Variance=1e-9  SampleTime=baseRate
  Calculated & Store Measured States : Subsystem
  Calculated & Store True States : Subsystem
  Coriolis Function1 : MATLAB Function  TreatAsAtomicUnit=on
  Data @ Measurement Rate : Subsystem
  Data Store Read3 : DataStoreRead  DataStoreName=ARM_Controls  IndexOptions=Index vector (dialog)  Indices=1  OutputSizes=1
  Delay : Delay  DelayLength=1
  Demux : Demux  Outputs=[1,1,10]
  Dynamics Model : MATLAB Function  TreatAsAtomicUnit=on
  Exceeded Table Limits : Subsystem
  Inertia Function 1 : MATLAB Function  TreatAsAtomicUnit=on
  Mux : Mux  Inputs=2
  Mux2 : Mux  Inputs=2
  Saturated Control Commands for RED : DataStoreRead  DataStoreName=RED_Saturated_Controls  IndexOptions=Index vector (dialog)  Indices=1  OutputSizes=1
  Stop Simulation : Stop
  Sum : Sum  Inputs=++|
  Terminator : Terminator
  Velocity to Position : DiscreteIntegrator  IntegratorMethod=Integration: Backward Euler  InitialCondition=[drop_states_RED,drop_states_ARM]  SampleTime=-1  ICPrevOutput=DiscIntNeverNeededParam  ICPrevScaledInput=DiscIntNeverNeededParam
  wires:
  Mux2/1 -> Dynamics Model/4(u)
  Data Store Read3/1 -> Mux2/2
  Dynamics Model/1(q_dot) -> Velocity to Position/1
  Coriolis Function1/1(CoriolisS) -> Dynamics Model/3(CoriolisS)
  Delay/1 -> Coriolis Function1/1(x), Inertia Function 1/1(x), Dynamics Model/1(x)
  Inertia Function 1/1(InertiaS) -> Dynamics Model/2(InertiaS)
  Saturated Control Commands for RED/1 -> Mux2/1
  Data @ Measurement Rate/2(Time Step) -> Calculated & Store Measured States/2(dt)
  Mux/1 -> Demux/1, Delay/1
  Dynamics Model/2(q_ddot) -> Acceleration to Velocity/1
  Acceleration to Velocity/1 -> Mux/2
  Demux/1 -> Exceeded Table Limits/1(X)
  Exceeded Table Limits/1(Stop) -> Stop Simulation/1
  Demux/2 -> Exceeded Table Limits/2(Y)
  Demux/3 -> Terminator/1
  Add Noise/1 -> Sum/1
  Velocity to Position/1 -> Sum/2, Calculated & Store True States/1(y), Mux/1
  Sum/1 -> Data @ Measurement Rate/1(Data Input)
  Data @ Measurement Rate/1(Data Held) -> Calculated & Store Measured States/1(y)

== system spot410/Simulate Plant Dynamics/RED and ARM Dynamics/RED Only ==
  Action Port : ActionPort  ActionPortLabel=else
  Add Noise : RandomNumber  Variance=1e-9  SampleTime=baseRate
  Calculated & Store Measured States : Subsystem
  Calculated & Store True States : Subsystem
  Data @ Measurement Rate : Subsystem
  Dynamics Model for RED : Subsystem  SystemSampleTime=serverRate
      settings: PortSchema="{\"entries\":[{\"content\":{\"sides\":[{\"content\":{\"connectorIds\":[\"In1\"]},\"type\":\"ConnectorPlacement.EquallySpacedRectSide\",\"uuid\":\"36f8472d-4371-4b5e-bb25-792dc7798e2d\"},{\"content\":{\"side\":\"RIGHT\"},\"type\":\"ConnectorPlacement.EquallySpacedRectSide\",\"uuid\":\"cd500640-3349-40a3-88e5-d39ca64affda\"},{\"content\":{\"connectorIds\":[\"Out1\"],\"side\":\"TOP\"},\"type\":\"ConnectorPlacement.EquallySpacedRectSide\",\"uuid\":\"f35070a8-6b00-4762-8673-30fcbcb2fe63\"}]},\"type\":\"ConnectorPlacement.EquallySpacedConnector\",\"uuid\":\"7478ab5e-be27-4ef2-a158-875ec93c8619\"}],\"packageUris\":[\"http://schema.mathworks.com/mf0/Connector/R2020b\"],\"version\":\"1.0\"}"
  Saturated Control Commands for RED : DataStoreRead  DataStoreName=RED_Saturated_Controls  IndexOptions=Index vector (dialog)  Indices=1  OutputSizes=1
  Sum : Sum  Inputs=++|
  wires:
  Saturated Control Commands for RED/1 -> Dynamics Model for RED/1(control_inputs)
  Data @ Measurement Rate/2(Time Step) -> Calculated & Store Measured States/2(dt)
  Data @ Measurement Rate/1(Data Held) -> Calculated & Store Measured States/1(y)
  Add Noise/1 -> Sum/1
  Dynamics Model for RED/1(states) -> Sum/2, Calculated & Store True States/1(y)
  Sum/1 -> Data @ Measurement Rate/1(Data Input)

== system spot410/Thruster Control Code/Change BLACK Behavior/Calculate Duty Cycle ==
  "[Fx_b; Fy_b; Tz]" : Inport
  Measured Attitude : Inport  Port=2
  Demux : Demux  Outputs=3
  Duty Cycle @ PWM : Subsystem
  Generate Initial Guess : Subsystem
  MATLAB Function1 : MATLAB Function  TreatAsAtomicUnit=on
  MATLAB Function5 : MATLAB Function  TreatAsAtomicUnit=on  mask{max_iters=1, tol=1e-3}
      mask prompts: max_iters "Maximum Number of Iterations"; tol "Convergence Tolerance"
  Mux : Mux  Inputs=2
  Mux1 : Mux  Inputs=2
  Product1 : Product  Multiplication=Matrix(*)
  Reshape : Reshape  OutputDimensionality=Column vector (2-D)
  Rotate Forces to Inertial : Subsystem
  Duty Cycle : Outport  VectorParamsAs1DForOutWhenUnconnected=off
  Saturated Forces Moments : Outport  Port=2
  wires:
  Rotate Forces to Inertial/1(F_I) -> Mux1/1
  Generate Initial Guess/1(Duty Cycle) -> MATLAB Function5/2(x0)
  Product1/1 -> Demux/1
  Measured Attitude/1 -> Rotate Forces to Inertial/2(Rz)
  Duty Cycle @ PWM/1(Duty Cycle Held) -> Product1/2
  "[Fx_b; Fy_b; Tz]"/1 -> Generate Initial Guess/1("[Fx; Fy; Tz]"), Reshape/1
  MATLAB Function5/2(duty_cycles) -> MATLAB Function1/1(ThrustPer), Duty Cycle/1
  Demux/2 -> Mux/2
  Mux/1 -> Rotate Forces to Inertial/1("F_b ")
  Demux/3 -> Mux1/2
  Demux/1 -> Mux/1
  Reshape/1 -> MATLAB Function5/1(u_desired)
  MATLAB Function5/1(H_final) -> Product1/1
  Mux1/1 -> Saturated Forces Moments/1
  MATLAB Function1/1(ThrustPer_Final) -> Duty Cycle @ PWM/1(ThrustPer_Final)

== system spot410/Thruster Control Code/Change BLACK Behavior/Rotate Forces to Body ==
  "F_I " : Inport
  Rz : Inport  Port=2
  Create Rotation Matrix : MATLAB Function  TreatAsAtomicUnit=on
  Rotate F_I to F_b : Product  Multiplication=Matrix(*)
  F_b : Outport  VectorParamsAs1DForOutWhenUnconnected=off
  wires:
  Rotate F_I to F_b/1 -> F_b/1
  Create Rotation Matrix/1(C_bI) -> Rotate F_I to F_b/1
  "F_I "/1 -> Rotate F_I to F_b/2
  Rz/1 -> Create Rotation Matrix/1(Rz)

== system spot410/Thruster Control Code/Change BLUE Behavior/Calculate Duty Cycle ==
  "[Fx_b; Fy_b; Tz]" : Inport
  Measured Attitude : Inport  Port=2
  Demux : Demux  Outputs=3
  Duty Cycle @ PWM : Subsystem
  Generate Initial Guess : Subsystem
  MATLAB Function1 : MATLAB Function  TreatAsAtomicUnit=on
  MATLAB Function5 : MATLAB Function  TreatAsAtomicUnit=on  mask{max_iters=1, tol=1e-3}
      mask prompts: max_iters "Maximum Number of Iterations"; tol "Convergence Tolerance"
  Mux : Mux  Inputs=2
  Mux1 : Mux  Inputs=2
  Product1 : Product  Multiplication=Matrix(*)
  Reshape : Reshape  OutputDimensionality=Column vector (2-D)
  Rotate Forces to Inertial : Subsystem
  Duty Cycle : Outport  VectorParamsAs1DForOutWhenUnconnected=off
  Saturated Forces Moments : Outport  Port=2
  wires:
  Rotate Forces to Inertial/1(F_I) -> Mux1/1
  Generate Initial Guess/1(Duty Cycle) -> MATLAB Function5/2(x0)
  Product1/1 -> Demux/1
  Measured Attitude/1 -> Rotate Forces to Inertial/2(Rz)
  Duty Cycle @ PWM/1(Duty Cycle Held) -> Product1/2
  "[Fx_b; Fy_b; Tz]"/1 -> Generate Initial Guess/1("[Fx; Fy; Tz]"), Reshape/1
  MATLAB Function5/2(duty_cycles) -> Duty Cycle/1, MATLAB Function1/1(ThrustPer)
  Demux/2 -> Mux/2
  Mux/1 -> Rotate Forces to Inertial/1("F_b ")
  Demux/3 -> Mux1/2
  Demux/1 -> Mux/1
  Reshape/1 -> MATLAB Function5/1(u_desired)
  Mux1/1 -> Saturated Forces Moments/1
  MATLAB Function5/1(H_final) -> Product1/1
  MATLAB Function1/1(ThrustPer_Final) -> Duty Cycle @ PWM/1(ThrustPer_Final)

== system spot410/Thruster Control Code/Change BLUE Behavior/Rotate Forces to Body ==
  "F_I " : Inport
  Rz : Inport  Port=2
  Create Rotation Matrix : MATLAB Function  TreatAsAtomicUnit=on
  Rotate F_I to F_b : Product  Multiplication=Matrix(*)
  F_b : Outport  VectorParamsAs1DForOutWhenUnconnected=off
  wires:
  Rotate F_I to F_b/1 -> F_b/1
  Create Rotation Matrix/1(C_bI) -> Rotate F_I to F_b/1
  "F_I "/1 -> Rotate F_I to F_b/2
  Rz/1 -> Create Rotation Matrix/1(Rz)

== system spot410/Thruster Control Code/Change RED Behavior/Calculate Duty Cycle ==
  "[Fx_b; Fy_b; Tz]" : Inport
  Measured Attitude : Inport  Port=2
  Demux : Demux  Outputs=3
  Duty Cycle @ PWM : Subsystem
  Generate Initial Guess : Subsystem
  MATLAB Function5 : MATLAB Function  TreatAsAtomicUnit=on  mask{max_iters=1, tol=1e-3}
      mask prompts: max_iters "Maximum Number of Iterations"; tol "Convergence Tolerance"
  MATLAB Function8 : MATLAB Function  TreatAsAtomicUnit=on
  Mux : Mux  Inputs=2
  Mux1 : Mux  Inputs=2
  Product1 : Product  Multiplication=Matrix(*)
  Reshape : Reshape  OutputDimensionality=Column vector (2-D)
  Rotate Forces to Inertial : Subsystem
  Duty Cycle : Outport  VectorParamsAs1DForOutWhenUnconnected=off
  Saturated Forces Moments : Outport  Port=2
  wires:
  Demux/2 -> Mux/2
  Measured Attitude/1 -> Rotate Forces to Inertial/2(Rz)
  Rotate Forces to Inertial/1(F_I) -> Mux1/1
  Product1/1 -> Demux/1
  Demux/1 -> Mux/1
  Mux/1 -> Rotate Forces to Inertial/1("F_b ")
  Demux/3 -> Mux1/2
  Reshape/1 -> MATLAB Function5/1(u_desired)
  MATLAB Function5/1(H_final) -> Product1/1
  MATLAB Function5/2(duty_cycles) -> Duty Cycle/1, MATLAB Function8/1(ThrustPer)
  Duty Cycle @ PWM/1(Duty Cycle Held) -> Product1/2
  Generate Initial Guess/1(Duty Cycle) -> MATLAB Function5/2(x0)
  "[Fx_b; Fy_b; Tz]"/1 -> Generate Initial Guess/1("[Fx; Fy; Tz]"), Reshape/1
  MATLAB Function8/1(ThrustPer_Final) -> Duty Cycle @ PWM/1(ThrustPer_Final)
  Mux1/1 -> Saturated Forces Moments/1

== system spot410/Thruster Control Code/Change RED Behavior/Rotate Forces to Body ==
  "F_I " : Inport
  Rz : Inport  Port=2
  Create Rotation Matrix : MATLAB Function  TreatAsAtomicUnit=on
  Rotate F_I to F_b : Product  Multiplication=Matrix(*)
  F_b : Outport  VectorParamsAs1DForOutWhenUnconnected=off
  wires:
  Rotate F_I to F_b/1 -> F_b/1
  Create Rotation Matrix/1(C_bI) -> Rotate F_I to F_b/1
  "F_I "/1 -> Rotate F_I to F_b/2
  Rz/1 -> Create Rotation Matrix/1(Rz)

== system spot410/1 - Experiment Logic/Phase #3: Experiment/Sub-Phase #1/Desired Joint Angles RED ==
  Constant1 : Constant  Value=pi/2
  Constant2 : Constant  Value=0
  Constant3 : Constant  Value=pi/2
  Mux : Mux  Inputs=3
  Target Array : Outport
  wires:
  Mux/1 -> Target Array/1
  Constant3/1 -> Mux/1
  Constant1/1 -> Mux/2
  Constant2/1 -> Mux/3
